simulink model "EHB_speedgoat_R2020a_V1"  (R2020a)
settings: Solver=FixedStepDiscrete  StartTime=0.0  StopTime=inf  FixedStep=0.001  RelTol=1e-3  EnableMultiTasking=on
model workspace (MAT data in the model file):
  A : Simulink.Signal (value not decoded)
  B : Simulink.Signal (value not decoded)
  C : Simulink.Signal (value not decoded)
  D : Simulink.Signal (value not decoded)
  E : Simulink.Signal (value not decoded)
  calin = [-9.96 -7.98 -5.98 -3.99 -1.994 0 1.995 3.992 5.99 7.98 9.97]
  calout = [-10 -8 -6 -4 -2 0 2 4 6 8 10]
symbols that are objects in the model workspace (value not decoded): C, D
undefined symbols (not defined in the file): Com1, none, ts_IO612
libraries: simulink x1436, xpcethercatlib x1223, yisutbxlib_utilities x256, xpcutilitieslib x156, hdlsllib x145, canmsglib x46, speedgoatlib_IO602_4 x11, speedgoatlib_IO611 x7, slrttcplib x4, CanManageLib x3, slrtlib x3, xpcseriallib x2
(part 5 of 30)

== system EHB_speedgoat_R2020a_V1/TIF_04/CB2020_3/Sw6 ==
  In2 : Inport
  In3 : Inport  Port=2
  Vol : Inport  Port=3
  Add : Sum
  Add1 : Sum
  Constant : Constant  Value=0.02
  Constant1 : Constant  Value=0.01
  Switch : Switch  Criteria=u2 > Threshold  Threshold=2.2
  Out1 : Outport
  wires:
  Constant/1 -> Add/2
  Add/1 -> Switch/3
  Add1/1 -> Switch/1
  Switch/1 -> Out1/1
  In3/1 -> Add/1
  In2/1 -> Switch/2
  Constant1/1 -> Add1/1
  Vol/1 -> Add1/2

== system EHB_speedgoat_R2020a_V1/TIF_04/CB2020_3/Sw7 ==
  In2 : Inport
  In3 : Inport  Port=2
  Vol : Inport  Port=3
  Add : Sum
  Add1 : Sum
  Constant : Constant  Value=0.02
  Constant1 : Constant  Value=0.01
  Switch : Switch  Criteria=u2 > Threshold  Threshold=2.2
  Out1 : Outport
  wires:
  In2/1 -> Switch/2
  In3/1 -> Add/1
  Switch/1 -> Out1/1
  Add1/1 -> Switch/1
  Add/1 -> Switch/3
  Constant/1 -> Add/2
  Constant1/1 -> Add1/1
  Vol/1 -> Add1/2

== system EHB_speedgoat_R2020a_V1/TIF_04/CB2020_3/Sw8 ==
  Vol : Inport
  In2 : Inport  Port=2
  In3 : Inport  Port=3
  Add : Sum
  Add1 : Sum
  Constant : Constant  Value=0.02
  Constant1 : Constant  Value=0.01
  Switch : Switch  Criteria=u2 > Threshold  Threshold=2.2
  Out1 : Outport
  wires:
  Constant/1 -> Add/2
  Add/1 -> Switch/3
  Switch/1 -> Out1/1
  In3/1 -> Add/1
  In2/1 -> Switch/2
  Constant1/1 -> Add1/1
  Vol/1 -> Add1/2
  Add1/1 -> Switch/1

== system EHB_speedgoat_R2020a_V1/TIF_04/CB2020_3/Sw9 ==
  In2 : Inport
  In3 : Inport  Port=2
  Vol : Inport  Port=3
  Add : Sum
  Add1 : Sum
  Constant : Constant  Value=0.02
  Constant1 : Constant  Value=0.01
  Switch : Switch  Criteria=u2 > Threshold  Threshold=2.2
  Out1 : Outport
  wires:
  In2/1 -> Switch/2
  In3/1 -> Add/1
  Switch/1 -> Out1/1
  Add1/1 -> Switch/1
  Add/1 -> Switch/3
  Constant/1 -> Add/2
  Constant1/1 -> Add1/1
  Vol/1 -> Add1/2

== system EHB_speedgoat_R2020a_V1/TIF_04/CB2020_3/mean1 ==
  In1 : Inport
  Add : Sum
  Add1 : Sum  Inputs=++++++++++++++++++++
  Add2 : Sum  Inputs=++++++++++++++++++++
  Delay{,1..39} (40 alike) : Delay  DelayLength=1
  Gain : Gain  Gain=1/40
  Vol : Outport
  wires:
  Add/1 -> Gain/1
  Gain/1 -> Vol/1
  Delay36/1 -> Delay37/1, Add2/7
  Delay37/1 -> Delay38/1, Add2/8
  Delay34/1 -> Delay35/1, Add2/5
  Delay33/1 -> Delay34/1, Add2/4
  Delay20/1 -> Delay21/1, Add2/1
  Delay32/1 -> Delay33/1, Add2/3
  Add2/1 -> Add/2
  Delay35/1 -> Delay36/1, Add2/6
  Delay21/1 -> Delay32/1, Add2/2
  Delay38/1 -> Delay39/1, Add2/9
  Delay39/1 -> Delay22/1, Add2/10
  Delay31/1 -> Add2/20
  Delay19/1 -> Add1/20, Delay20/1
  Delay30/1 -> Delay31/1, Add2/19
  Delay23/1 -> Delay24/1, Add2/12
  Delay27/1 -> Delay28/1, Add2/16
  Delay24/1 -> Delay25/1, Add2/13
  Delay22/1 -> Delay23/1, Add2/11
  Delay25/1 -> Delay26/1, Add2/14
  Delay26/1 -> Delay27/1, Add2/15
  Delay29/1 -> Delay30/1, Add2/18
  Delay28/1 -> Delay29/1, Add2/17
  Delay16/1 -> Add1/17, Delay17/1
  Delay17/1 -> Add1/18, Delay18/1
  Delay14/1 -> Add1/15, Delay15/1
  Delay13/1 -> Add1/14, Delay14/1
  Delay10/1 -> Add1/11, Delay11/1
  Delay12/1 -> Add1/13, Delay13/1
  Delay15/1 -> Add1/16, Delay16/1
  Delay11/1 -> Add1/12, Delay12/1
  Delay18/1 -> Add1/19, Delay19/1
  In1/1 -> Delay/1
  Delay9/1 -> Add1/10, Delay10/1
  Delay8/1 -> Add1/9, Delay9/1
  Delay1/1 -> Add1/2, Delay2/1
  Delay5/1 -> Add1/6, Delay6/1
  Add1/1 -> Add/1
  Delay2/1 -> Add1/3, Delay3/1
  Delay/1 -> Add1/1, Delay1/1
  Delay3/1 -> Add1/4, Delay4/1
  Delay4/1 -> Add1/5, Delay5/1
  Delay7/1 -> Add1/8, Delay8/1
  Delay6/1 -> Add1/7, Delay7/1

== system EHB_speedgoat_R2020a_V1/TIF_04/CB2020_3/mean10 ==
  In1 : Inport
  Add : Sum
  Add1 : Sum  Inputs=++++++++++++++++++++
  Add2 : Sum  Inputs=++++++++++++++++++++
  Delay{,1..39} (40 alike) : Delay  DelayLength=1
  Gain : Gain  Gain=1/40
  Vol : Outport
  wires:
  Delay6/1 -> Delay7/1, Add1/7
  Delay7/1 -> Delay8/1, Add1/8
  Delay4/1 -> Delay5/1, Add1/5
  Delay3/1 -> Delay4/1, Add1/4
  Delay/1 -> Delay1/1, Add1/1
  Delay2/1 -> Delay3/1, Add1/3
  Add1/1 -> Add/1
  Delay5/1 -> Delay6/1, Add1/6
  Delay1/1 -> Delay2/1, Add1/2
  Delay8/1 -> Delay9/1, Add1/9
  Delay9/1 -> Delay10/1, Add1/10
  In1/1 -> Delay/1
  Delay18/1 -> Delay19/1, Add1/19
  Delay11/1 -> Delay12/1, Add1/12
  Delay15/1 -> Delay16/1, Add1/16
  Delay12/1 -> Delay13/1, Add1/13
  Delay10/1 -> Delay11/1, Add1/11
  Delay13/1 -> Delay14/1, Add1/14
  Delay14/1 -> Delay15/1, Add1/15
  Delay17/1 -> Delay18/1, Add1/18
  Delay16/1 -> Delay17/1, Add1/17
  Delay28/1 -> Add2/17, Delay29/1
  Delay29/1 -> Add2/18, Delay30/1
  Delay26/1 -> Add2/15, Delay27/1
  Delay25/1 -> Add2/14, Delay26/1
  Delay22/1 -> Add2/11, Delay23/1
  Delay24/1 -> Add2/13, Delay25/1
  Delay27/1 -> Add2/16, Delay28/1
  Delay23/1 -> Add2/12, Delay24/1
  Delay30/1 -> Add2/19, Delay31/1
  Delay19/1 -> Delay20/1, Add1/20
  Delay31/1 -> Add2/20
  Delay39/1 -> Add2/10, Delay22/1
  Delay38/1 -> Add2/9, Delay39/1
  Delay21/1 -> Add2/2, Delay32/1
  Delay35/1 -> Add2/6, Delay36/1
  Add2/1 -> Add/2
  Delay32/1 -> Add2/3, Delay33/1
  Delay20/1 -> Add2/1, Delay21/1
  Delay33/1 -> Add2/4, Delay34/1
  Delay34/1 -> Add2/5, Delay35/1
  Delay37/1 -> Add2/8, Delay38/1
  Delay36/1 -> Add2/7, Delay37/1
  Gain/1 -> Vol/1
  Add/1 -> Gain/1

== system EHB_speedgoat_R2020a_V1/TIF_04/CB2020_3/mean11 ==
  In1 : Inport
  Add : Sum
  Add1 : Sum  Inputs=++++++++++++++++++++
  Add2 : Sum  Inputs=++++++++++++++++++++
  Delay{,1..39} (40 alike) : Delay  DelayLength=1
  Gain : Gain  Gain=1/40
  Vol : Outport
  wires:
  Add/1 -> Gain/1
  Gain/1 -> Vol/1
  Delay36/1 -> Delay37/1, Add2/7
  Delay37/1 -> Delay38/1, Add2/8
  Delay34/1 -> Delay35/1, Add2/5
  Delay33/1 -> Delay34/1, Add2/4
  Delay20/1 -> Delay21/1, Add2/1
  Delay32/1 -> Delay33/1, Add2/3
  Add2/1 -> Add/2
  Delay35/1 -> Delay36/1, Add2/6
  Delay21/1 -> Delay32/1, Add2/2
  Delay38/1 -> Delay39/1, Add2/9
  Delay39/1 -> Delay22/1, Add2/10
  Delay31/1 -> Add2/20
  Delay19/1 -> Add1/20, Delay20/1
  Delay30/1 -> Delay31/1, Add2/19
  Delay23/1 -> Delay24/1, Add2/12
  Delay27/1 -> Delay28/1, Add2/16
  Delay24/1 -> Delay25/1, Add2/13
  Delay22/1 -> Delay23/1, Add2/11
  Delay25/1 -> Delay26/1, Add2/14
  Delay26/1 -> Delay27/1, Add2/15
  Delay29/1 -> Delay30/1, Add2/18
  Delay28/1 -> Delay29/1, Add2/17
  Delay16/1 -> Add1/17, Delay17/1
  Delay17/1 -> Add1/18, Delay18/1
  Delay14/1 -> Add1/15, Delay15/1
  Delay13/1 -> Add1/14, Delay14/1
  Delay10/1 -> Add1/11, Delay11/1
  Delay12/1 -> Add1/13, Delay13/1
  Delay15/1 -> Add1/16, Delay16/1
  Delay11/1 -> Add1/12, Delay12/1
  Delay18/1 -> Add1/19, Delay19/1
  In1/1 -> Delay/1
  Delay9/1 -> Add1/10, Delay10/1
  Delay8/1 -> Add1/9, Delay9/1
  Delay1/1 -> Add1/2, Delay2/1
  Delay5/1 -> Add1/6, Delay6/1
  Add1/1 -> Add/1
  Delay2/1 -> Add1/3, Delay3/1
  Delay/1 -> Add1/1, Delay1/1
  Delay3/1 -> Add1/4, Delay4/1
  Delay4/1 -> Add1/5, Delay5/1
  Delay7/1 -> Add1/8, Delay8/1
  Delay6/1 -> Add1/7, Delay7/1

== system EHB_speedgoat_R2020a_V1/TIF_04/CB2020_3/mean12 ==
  In1 : Inport
  Add : Sum
  Add1 : Sum  Inputs=++++++++++++++++++++
  Add2 : Sum  Inputs=++++++++++++++++++++
  Delay{,1..39} (40 alike) : Delay  DelayLength=1
  Gain : Gain  Gain=1/40
  Vol : Outport
  wires:
  Delay6/1 -> Delay7/1, Add1/7
  Delay7/1 -> Delay8/1, Add1/8
  Delay4/1 -> Delay5/1, Add1/5
  Delay3/1 -> Delay4/1, Add1/4
  Delay/1 -> Delay1/1, Add1/1
  Delay2/1 -> Delay3/1, Add1/3
  Add1/1 -> Add/1
  Delay5/1 -> Delay6/1, Add1/6
  Delay1/1 -> Delay2/1, Add1/2
  Delay8/1 -> Delay9/1, Add1/9
  Delay9/1 -> Delay10/1, Add1/10
  In1/1 -> Delay/1
  Delay18/1 -> Delay19/1, Add1/19
  Delay11/1 -> Delay12/1, Add1/12
  Delay15/1 -> Delay16/1, Add1/16
  Delay12/1 -> Delay13/1, Add1/13
  Delay10/1 -> Delay11/1, Add1/11
  Delay13/1 -> Delay14/1, Add1/14
  Delay14/1 -> Delay15/1, Add1/15
  Delay17/1 -> Delay18/1, Add1/18
  Delay16/1 -> Delay17/1, Add1/17
  Delay28/1 -> Add2/17, Delay29/1
  Delay29/1 -> Add2/18, Delay30/1
  Delay26/1 -> Add2/15, Delay27/1
  Delay25/1 -> Add2/14, Delay26/1
  Delay22/1 -> Add2/11, Delay23/1
  Delay24/1 -> Add2/13, Delay25/1
  Delay27/1 -> Add2/16, Delay28/1
  Delay23/1 -> Add2/12, Delay24/1
  Delay30/1 -> Add2/19, Delay31/1
  Delay19/1 -> Delay20/1, Add1/20
  Delay31/1 -> Add2/20
  Delay39/1 -> Add2/10, Delay22/1
  Delay38/1 -> Add2/9, Delay39/1
  Delay21/1 -> Add2/2, Delay32/1
  Delay35/1 -> Add2/6, Delay36/1
  Add2/1 -> Add/2
  Delay32/1 -> Add2/3, Delay33/1
  Delay20/1 -> Add2/1, Delay21/1
  Delay33/1 -> Add2/4, Delay34/1
  Delay34/1 -> Add2/5, Delay35/1
  Delay37/1 -> Add2/8, Delay38/1
  Delay36/1 -> Add2/7, Delay37/1
  Gain/1 -> Vol/1
  Add/1 -> Gain/1

== system EHB_speedgoat_R2020a_V1/TIF_04/CB2020_3/mean13 ==
  In1 : Inport
  Add : Sum  Inputs=++++
  Add{1..4} (4 alike) : Sum  Inputs=++++++++++++++++++++
  Delay{,1..79} (80 alike) : Delay  DelayLength=1
  Gain : Gain  Gain=1/80
  Vol : Outport
  wires:
  Add/1 -> Gain/1
  Gain/1 -> Vol/1
  Delay36/1 -> Delay37/1, Add2/7
  Delay37/1 -> Delay38/1, Add2/8
  Delay34/1 -> Delay35/1, Add2/5
  Delay33/1 -> Delay34/1, Add2/4
  Delay20/1 -> Delay21/1, Add2/1
  Delay32/1 -> Delay33/1, Add2/3
  Add2/1 -> Add/2
  Delay35/1 -> Delay36/1, Add2/6
  Delay21/1 -> Delay32/1, Add2/2
  Delay38/1 -> Delay39/1, Add2/9
  Delay39/1 -> Delay22/1, Add2/10
  Delay19/1 -> Add1/20, Delay20/1
  Delay30/1 -> Delay31/1, Add2/19
  Delay23/1 -> Delay24/1, Add2/12
  Delay27/1 -> Delay28/1, Add2/16
  Delay24/1 -> Delay25/1, Add2/13
  Delay22/1 -> Delay23/1, Add2/11
  Delay25/1 -> Delay26/1, Add2/14
  Delay26/1 -> Delay27/1, Add2/15
  Delay29/1 -> Delay30/1, Add2/18
  Delay28/1 -> Delay29/1, Add2/17
  Delay16/1 -> Add1/17, Delay17/1
  Delay17/1 -> Add1/18, Delay18/1
  Delay14/1 -> Add1/15, Delay15/1
  Delay13/1 -> Add1/14, Delay14/1
  Delay10/1 -> Add1/11, Delay11/1
  Delay12/1 -> Add1/13, Delay13/1
  Delay15/1 -> Add1/16, Delay16/1
  Delay11/1 -> Add1/12, Delay12/1
  Delay18/1 -> Add1/19, Delay19/1
  In1/1 -> Delay/1
  Delay9/1 -> Add1/10, Delay10/1
  Delay8/1 -> Add1/9, Delay9/1
  Delay1/1 -> Add1/2, Delay2/1
  Delay5/1 -> Add1/6, Delay6/1
  Add1/1 -> Add/1
  Delay2/1 -> Add1/3, Delay3/1
  Delay/1 -> Add1/1, Delay1/1
  Delay3/1 -> Add1/4, Delay4/1
  Delay4/1 -> Add1/5, Delay5/1
  Delay7/1 -> Add1/8, Delay8/1
  Delay6/1 -> Add1/7, Delay7/1
  Delay48/1 -> Add3/17, Delay49/1
  Delay49/1 -> Add3/18, Delay50/1
  Delay46/1 -> Add3/15, Delay47/1
  Delay45/1 -> Add3/14, Delay46/1
  Delay42/1 -> Add3/11, Delay43/1
  Delay44/1 -> Add3/13, Delay45/1
  Delay47/1 -> Add3/16, Delay48/1
  Delay43/1 -> Add3/12, Delay44/1
  Delay50/1 -> Add3/19, Delay51/1
  Delay31/1 -> Delay40/1, Add2/20
  Delay59/1 -> Add3/10, Delay42/1
  Delay58/1 -> Add3/9, Delay59/1
  Delay41/1 -> Add3/2, Delay52/1
  Delay55/1 -> Add3/6, Delay56/1
  Add3/1 -> Add/3
  Delay52/1 -> Add3/3, Delay53/1
  Delay40/1 -> Add3/1, Delay41/1
  Delay53/1 -> Add3/4, Delay54/1
  Delay54/1 -> Add3/5, Delay55/1
  Delay57/1 -> Add3/8, Delay58/1
  Delay56/1 -> Add3/7, Delay57/1
  Delay76/1 -> Delay77/1, Add4/7
  Delay77/1 -> Delay78/1, Add4/8
  Delay74/1 -> Delay75/1, Add4/5
  Delay73/1 -> Delay74/1, Add4/4
  Delay60/1 -> Delay61/1, Add4/1
  Delay72/1 -> Delay73/1, Add4/3
  Add4/1 -> Add/4
  Delay75/1 -> Delay76/1, Add4/6
  Delay61/1 -> Delay72/1, Add4/2
  Delay78/1 -> Delay79/1, Add4/9
  Delay79/1 -> Delay62/1, Add4/10
  Delay71/1 -> Add4/20
  Delay51/1 -> Delay60/1, Add3/20
  Delay70/1 -> Delay71/1, Add4/19
  Delay63/1 -> Delay64/1, Add4/12
  Delay67/1 -> Delay68/1, Add4/16
  Delay64/1 -> Delay65/1, Add4/13
  Delay62/1 -> Delay63/1, Add4/11
  Delay65/1 -> Delay66/1, Add4/14
  Delay66/1 -> Delay67/1, Add4/15
  Delay69/1 -> Delay70/1, Add4/18
  Delay68/1 -> Delay69/1, Add4/17

== system EHB_speedgoat_R2020a_V1/TIF_04/CB2020_3/mean14 ==
  In1 : Inport
  Add : Sum  Inputs=++++
  Add{1..4} (4 alike) : Sum  Inputs=++++++++++++++++++++
  Delay{,1..79} (80 alike) : Delay  DelayLength=1
  Gain : Gain  Gain=1/80
  Vol : Outport
  wires:
  Delay68/1 -> Add4/17, Delay69/1
  Delay69/1 -> Add4/18, Delay70/1
  Delay66/1 -> Add4/15, Delay67/1
  Delay65/1 -> Add4/14, Delay66/1
  Delay62/1 -> Add4/11, Delay63/1
  Delay64/1 -> Add4/13, Delay65/1
  Delay67/1 -> Add4/16, Delay68/1
  Delay63/1 -> Add4/12, Delay64/1
  Delay70/1 -> Add4/19, Delay71/1
  Delay51/1 -> Add3/20, Delay60/1
  Delay71/1 -> Add4/20
  Delay79/1 -> Add4/10, Delay62/1
  Delay78/1 -> Add4/9, Delay79/1
  Delay61/1 -> Add4/2, Delay72/1
  Delay75/1 -> Add4/6, Delay76/1
  Add4/1 -> Add/4
  Delay72/1 -> Add4/3, Delay73/1
  Delay60/1 -> Add4/1, Delay61/1
  Delay73/1 -> Add4/4, Delay74/1
  Delay74/1 -> Add4/5, Delay75/1
  Delay77/1 -> Add4/8, Delay78/1
  Delay76/1 -> Add4/7, Delay77/1
  Delay56/1 -> Delay57/1, Add3/7
  Delay57/1 -> Delay58/1, Add3/8
  Delay54/1 -> Delay55/1, Add3/5
  Delay53/1 -> Delay54/1, Add3/4
  Delay40/1 -> Delay41/1, Add3/1
  Delay52/1 -> Delay53/1, Add3/3
  Add3/1 -> Add/3
  Delay55/1 -> Delay56/1, Add3/6
  Delay41/1 -> Delay52/1, Add3/2
  Delay58/1 -> Delay59/1, Add3/9
  Delay59/1 -> Delay42/1, Add3/10
  Delay31/1 -> Add2/20, Delay40/1
  Delay50/1 -> Delay51/1, Add3/19
  Delay43/1 -> Delay44/1, Add3/12
  Delay47/1 -> Delay48/1, Add3/16
  Delay44/1 -> Delay45/1, Add3/13
  Delay42/1 -> Delay43/1, Add3/11
  Delay45/1 -> Delay46/1, Add3/14
  Delay46/1 -> Delay47/1, Add3/15
  Delay49/1 -> Delay50/1, Add3/18
  Delay48/1 -> Delay49/1, Add3/17
  Delay6/1 -> Delay7/1, Add1/7
  Delay7/1 -> Delay8/1, Add1/8
  Delay4/1 -> Delay5/1, Add1/5
  Delay3/1 -> Delay4/1, Add1/4
  Delay/1 -> Delay1/1, Add1/1
  Delay2/1 -> Delay3/1, Add1/3
  Add1/1 -> Add/1
  Delay5/1 -> Delay6/1, Add1/6
  Delay1/1 -> Delay2/1, Add1/2
  Delay8/1 -> Delay9/1, Add1/9
  Delay9/1 -> Delay10/1, Add1/10
  In1/1 -> Delay/1
  Delay18/1 -> Delay19/1, Add1/19
  Delay11/1 -> Delay12/1, Add1/12
  Delay15/1 -> Delay16/1, Add1/16
  Delay12/1 -> Delay13/1, Add1/13
  Delay10/1 -> Delay11/1, Add1/11
  Delay13/1 -> Delay14/1, Add1/14
  Delay14/1 -> Delay15/1, Add1/15
  Delay17/1 -> Delay18/1, Add1/18
  Delay16/1 -> Delay17/1, Add1/17
  Delay28/1 -> Add2/17, Delay29/1
  Delay29/1 -> Add2/18, Delay30/1
  Delay26/1 -> Add2/15, Delay27/1
  Delay25/1 -> Add2/14, Delay26/1
  Delay22/1 -> Add2/11, Delay23/1
  Delay24/1 -> Add2/13, Delay25/1
  Delay27/1 -> Add2/16, Delay28/1
  Delay23/1 -> Add2/12, Delay24/1
  Delay30/1 -> Add2/19, Delay31/1
  Delay19/1 -> Delay20/1, Add1/20
  Delay39/1 -> Add2/10, Delay22/1
  Delay38/1 -> Add2/9, Delay39/1
  Delay21/1 -> Add2/2, Delay32/1
  Delay35/1 -> Add2/6, Delay36/1
  Add2/1 -> Add/2
  Delay32/1 -> Add2/3, Delay33/1
  Delay20/1 -> Add2/1, Delay21/1
  Delay33/1 -> Add2/4, Delay34/1
  Delay34/1 -> Add2/5, Delay35/1
  Delay37/1 -> Add2/8, Delay38/1
  Delay36/1 -> Add2/7, Delay37/1
  Gain/1 -> Vol/1
  Add/1 -> Gain/1

== system EHB_speedgoat_R2020a_V1/TIF_04/CB2020_3/mean15 ==
  In1 : Inport
  Add : Sum  Inputs=++++
  Add{1..4} (4 alike) : Sum  Inputs=++++++++++++++++++++
  Delay{,1..79} (80 alike) : Delay  DelayLength=1
  Gain : Gain  Gain=1/80
  Vol : Outport
  wires:
  Add/1 -> Gain/1
  Gain/1 -> Vol/1
  Delay36/1 -> Delay37/1, Add2/7
  Delay37/1 -> Delay38/1, Add2/8
  Delay34/1 -> Delay35/1, Add2/5
  Delay33/1 -> Delay34/1, Add2/4
  Delay20/1 -> Delay21/1, Add2/1
  Delay32/1 -> Delay33/1, Add2/3
  Add2/1 -> Add/2
  Delay35/1 -> Delay36/1, Add2/6
  Delay21/1 -> Delay32/1, Add2/2
  Delay38/1 -> Delay39/1, Add2/9
  Delay39/1 -> Delay22/1, Add2/10
  Delay19/1 -> Add1/20, Delay20/1
  Delay30/1 -> Delay31/1, Add2/19
  Delay23/1 -> Delay24/1, Add2/12
  Delay27/1 -> Delay28/1, Add2/16
  Delay24/1 -> Delay25/1, Add2/13
  Delay22/1 -> Delay23/1, Add2/11
  Delay25/1 -> Delay26/1, Add2/14
  Delay26/1 -> Delay27/1, Add2/15
  Delay29/1 -> Delay30/1, Add2/18
  Delay28/1 -> Delay29/1, Add2/17
  Delay16/1 -> Add1/17, Delay17/1
  Delay17/1 -> Add1/18, Delay18/1
  Delay14/1 -> Add1/15, Delay15/1
  Delay13/1 -> Add1/14, Delay14/1
  Delay10/1 -> Add1/11, Delay11/1
  Delay12/1 -> Add1/13, Delay13/1
  Delay15/1 -> Add1/16, Delay16/1
  Delay11/1 -> Add1/12, Delay12/1
  Delay18/1 -> Add1/19, Delay19/1
  In1/1 -> Delay/1
  Delay9/1 -> Add1/10, Delay10/1
  Delay8/1 -> Add1/9, Delay9/1
  Delay1/1 -> Add1/2, Delay2/1
  Delay5/1 -> Add1/6, Delay6/1
  Add1/1 -> Add/1
  Delay2/1 -> Add1/3, Delay3/1
  Delay/1 -> Add1/1, Delay1/1
  Delay3/1 -> Add1/4, Delay4/1
  Delay4/1 -> Add1/5, Delay5/1
  Delay7/1 -> Add1/8, Delay8/1
  Delay6/1 -> Add1/7, Delay7/1
  Delay48/1 -> Add3/17, Delay49/1
  Delay49/1 -> Add3/18, Delay50/1
  Delay46/1 -> Add3/15, Delay47/1
  Delay45/1 -> Add3/14, Delay46/1
  Delay42/1 -> Add3/11, Delay43/1
  Delay44/1 -> Add3/13, Delay45/1
  Delay47/1 -> Add3/16, Delay48/1
  Delay43/1 -> Add3/12, Delay44/1
  Delay50/1 -> Add3/19, Delay51/1
  Delay31/1 -> Delay40/1, Add2/20
  Delay59/1 -> Add3/10, Delay42/1
  Delay58/1 -> Add3/9, Delay59/1
  Delay41/1 -> Add3/2, Delay52/1
  Delay55/1 -> Add3/6, Delay56/1
  Add3/1 -> Add/3
  Delay52/1 -> Add3/3, Delay53/1
  Delay40/1 -> Add3/1, Delay41/1
  Delay53/1 -> Add3/4, Delay54/1
  Delay54/1 -> Add3/5, Delay55/1
  Delay57/1 -> Add3/8, Delay58/1
  Delay56/1 -> Add3/7, Delay57/1
  Delay76/1 -> Delay77/1, Add4/7
  Delay77/1 -> Delay78/1, Add4/8
  Delay74/1 -> Delay75/1, Add4/5
  Delay73/1 -> Delay74/1, Add4/4
  Delay60/1 -> Delay61/1, Add4/1
  Delay72/1 -> Delay73/1, Add4/3
  Add4/1 -> Add/4
  Delay75/1 -> Delay76/1, Add4/6
  Delay61/1 -> Delay72/1, Add4/2
  Delay78/1 -> Delay79/1, Add4/9
  Delay79/1 -> Delay62/1, Add4/10
  Delay71/1 -> Add4/20
  Delay51/1 -> Delay60/1, Add3/20
  Delay70/1 -> Delay71/1, Add4/19
  Delay63/1 -> Delay64/1, Add4/12
  Delay67/1 -> Delay68/1, Add4/16
  Delay64/1 -> Delay65/1, Add4/13
  Delay62/1 -> Delay63/1, Add4/11
  Delay65/1 -> Delay66/1, Add4/14
  Delay66/1 -> Delay67/1, Add4/15
  Delay69/1 -> Delay70/1, Add4/18
  Delay68/1 -> Delay69/1, Add4/17

== system EHB_speedgoat_R2020a_V1/TIF_04/CB2020_3/mean16 ==
  In1 : Inport
  Add : Sum  Inputs=++++
  Add{1..4} (4 alike) : Sum  Inputs=++++++++++++++++++++
  Delay{,1..79} (80 alike) : Delay  DelayLength=1
  Gain : Gain  Gain=1/80
  Vol : Outport
  wires:
  Delay68/1 -> Add4/17, Delay69/1
  Delay69/1 -> Add4/18, Delay70/1
  Delay66/1 -> Add4/15, Delay67/1
  Delay65/1 -> Add4/14, Delay66/1
  Delay62/1 -> Add4/11, Delay63/1
  Delay64/1 -> Add4/13, Delay65/1
  Delay67/1 -> Add4/16, Delay68/1
  Delay63/1 -> Add4/12, Delay64/1
  Delay70/1 -> Add4/19, Delay71/1
  Delay51/1 -> Add3/20, Delay60/1
  Delay71/1 -> Add4/20
  Delay79/1 -> Add4/10, Delay62/1
  Delay78/1 -> Add4/9, Delay79/1
  Delay61/1 -> Add4/2, Delay72/1
  Delay75/1 -> Add4/6, Delay76/1
  Add4/1 -> Add/4
  Delay72/1 -> Add4/3, Delay73/1
  Delay60/1 -> Add4/1, Delay61/1
  Delay73/1 -> Add4/4, Delay74/1
  Delay74/1 -> Add4/5, Delay75/1
  Delay77/1 -> Add4/8, Delay78/1
  Delay76/1 -> Add4/7, Delay77/1
  Delay56/1 -> Delay57/1, Add3/7
  Delay57/1 -> Delay58/1, Add3/8
  Delay54/1 -> Delay55/1, Add3/5
  Delay53/1 -> Delay54/1, Add3/4
  Delay40/1 -> Delay41/1, Add3/1
  Delay52/1 -> Delay53/1, Add3/3
  Add3/1 -> Add/3
  Delay55/1 -> Delay56/1, Add3/6
  Delay41/1 -> Delay52/1, Add3/2
  Delay58/1 -> Delay59/1, Add3/9
  Delay59/1 -> Delay42/1, Add3/10
  Delay31/1 -> Add2/20, Delay40/1
  Delay50/1 -> Delay51/1, Add3/19
  Delay43/1 -> Delay44/1, Add3/12
  Delay47/1 -> Delay48/1, Add3/16
  Delay44/1 -> Delay45/1, Add3/13
  Delay42/1 -> Delay43/1, Add3/11
  Delay45/1 -> Delay46/1, Add3/14
  Delay46/1 -> Delay47/1, Add3/15
  Delay49/1 -> Delay50/1, Add3/18
  Delay48/1 -> Delay49/1, Add3/17
  Delay6/1 -> Delay7/1, Add1/7
  Delay7/1 -> Delay8/1, Add1/8
  Delay4/1 -> Delay5/1, Add1/5
  Delay3/1 -> Delay4/1, Add1/4
  Delay/1 -> Delay1/1, Add1/1
  Delay2/1 -> Delay3/1, Add1/3
  Add1/1 -> Add/1
  Delay5/1 -> Delay6/1, Add1/6
  Delay1/1 -> Delay2/1, Add1/2
  Delay8/1 -> Delay9/1, Add1/9
  Delay9/1 -> Delay10/1, Add1/10
  In1/1 -> Delay/1
  Delay18/1 -> Delay19/1, Add1/19
  Delay11/1 -> Delay12/1, Add1/12
  Delay15/1 -> Delay16/1, Add1/16
  Delay12/1 -> Delay13/1, Add1/13
  Delay10/1 -> Delay11/1, Add1/11
  Delay13/1 -> Delay14/1, Add1/14
  Delay14/1 -> Delay15/1, Add1/15
  Delay17/1 -> Delay18/1, Add1/18
  Delay16/1 -> Delay17/1, Add1/17
  Delay28/1 -> Add2/17, Delay29/1
  Delay29/1 -> Add2/18, Delay30/1
  Delay26/1 -> Add2/15, Delay27/1
  Delay25/1 -> Add2/14, Delay26/1
  Delay22/1 -> Add2/11, Delay23/1
  Delay24/1 -> Add2/13, Delay25/1
  Delay27/1 -> Add2/16, Delay28/1
  Delay23/1 -> Add2/12, Delay24/1
  Delay30/1 -> Add2/19, Delay31/1
  Delay19/1 -> Delay20/1, Add1/20
  Delay39/1 -> Add2/10, Delay22/1
  Delay38/1 -> Add2/9, Delay39/1
  Delay21/1 -> Add2/2, Delay32/1
  Delay35/1 -> Add2/6, Delay36/1
  Add2/1 -> Add/2
  Delay32/1 -> Add2/3, Delay33/1
  Delay20/1 -> Add2/1, Delay21/1
  Delay33/1 -> Add2/4, Delay34/1
  Delay34/1 -> Add2/5, Delay35/1
  Delay37/1 -> Add2/8, Delay38/1
  Delay36/1 -> Add2/7, Delay37/1
  Gain/1 -> Vol/1
  Add/1 -> Gain/1

== system EHB_speedgoat_R2020a_V1/TIF_04/CB2020_3/mean2 ==
  In1 : Inport
  Add : Sum
  Add1 : Sum  Inputs=++++++++++++++++++++
  Add2 : Sum  Inputs=++++++++++++++++++++
  Delay{,1..39} (40 alike) : Delay  DelayLength=1
  Gain : Gain  Gain=1/40
  Vol : Outport
  wires:
  Delay6/1 -> Delay7/1, Add1/7
  Delay7/1 -> Delay8/1, Add1/8
  Delay4/1 -> Delay5/1, Add1/5
  Delay3/1 -> Delay4/1, Add1/4
  Delay/1 -> Delay1/1, Add1/1
  Delay2/1 -> Delay3/1, Add1/3
  Add1/1 -> Add/1
  Delay5/1 -> Delay6/1, Add1/6
  Delay1/1 -> Delay2/1, Add1/2
  Delay8/1 -> Delay9/1, Add1/9
  Delay9/1 -> Delay10/1, Add1/10
  In1/1 -> Delay/1
  Delay18/1 -> Delay19/1, Add1/19
  Delay11/1 -> Delay12/1, Add1/12
  Delay15/1 -> Delay16/1, Add1/16
  Delay12/1 -> Delay13/1, Add1/13
  Delay10/1 -> Delay11/1, Add1/11
  Delay13/1 -> Delay14/1, Add1/14
  Delay14/1 -> Delay15/1, Add1/15
  Delay17/1 -> Delay18/1, Add1/18
  Delay16/1 -> Delay17/1, Add1/17
  Delay28/1 -> Add2/17, Delay29/1
  Delay29/1 -> Add2/18, Delay30/1
  Delay26/1 -> Add2/15, Delay27/1
  Delay25/1 -> Add2/14, Delay26/1
  Delay22/1 -> Add2/11, Delay23/1
  Delay24/1 -> Add2/13, Delay25/1
  Delay27/1 -> Add2/16, Delay28/1
  Delay23/1 -> Add2/12, Delay24/1
  Delay30/1 -> Add2/19, Delay31/1
  Delay19/1 -> Delay20/1, Add1/20
  Delay31/1 -> Add2/20
  Delay39/1 -> Add2/10, Delay22/1
  Delay38/1 -> Add2/9, Delay39/1
  Delay21/1 -> Add2/2, Delay32/1
  Delay35/1 -> Add2/6, Delay36/1
  Add2/1 -> Add/2
  Delay32/1 -> Add2/3, Delay33/1
  Delay20/1 -> Add2/1, Delay21/1
  Delay33/1 -> Add2/4, Delay34/1
  Delay34/1 -> Add2/5, Delay35/1
  Delay37/1 -> Add2/8, Delay38/1
  Delay36/1 -> Add2/7, Delay37/1
  Gain/1 -> Vol/1
  Add/1 -> Gain/1

== system EHB_speedgoat_R2020a_V1/TIF_04/CB2020_3/mean3 ==
  In1 : Inport
  Add : Sum
  Add1 : Sum  Inputs=++++++++++++++++++++
  Add2 : Sum  Inputs=++++++++++++++++++++
  Delay{,1..39} (40 alike) : Delay  DelayLength=1
  Gain : Gain  Gain=1/40
  Vol : Outport
  wires:
  Add/1 -> Gain/1
  Gain/1 -> Vol/1
  Delay36/1 -> Delay37/1, Add2/7
  Delay37/1 -> Delay38/1, Add2/8
  Delay34/1 -> Delay35/1, Add2/5
  Delay33/1 -> Delay34/1, Add2/4
  Delay20/1 -> Delay21/1, Add2/1
  Delay32/1 -> Delay33/1, Add2/3
  Add2/1 -> Add/2
  Delay35/1 -> Delay36/1, Add2/6
  Delay21/1 -> Delay32/1, Add2/2
  Delay38/1 -> Delay39/1, Add2/9
  Delay39/1 -> Delay22/1, Add2/10
  Delay31/1 -> Add2/20
  Delay19/1 -> Add1/20, Delay20/1
  Delay30/1 -> Delay31/1, Add2/19
  Delay23/1 -> Delay24/1, Add2/12
  Delay27/1 -> Delay28/1, Add2/16
  Delay24/1 -> Delay25/1, Add2/13
  Delay22/1 -> Delay23/1, Add2/11
  Delay25/1 -> Delay26/1, Add2/14
  Delay26/1 -> Delay27/1, Add2/15
  Delay29/1 -> Delay30/1, Add2/18
  Delay28/1 -> Delay29/1, Add2/17
  Delay16/1 -> Add1/17, Delay17/1
  Delay17/1 -> Add1/18, Delay18/1
  Delay14/1 -> Add1/15, Delay15/1
  Delay13/1 -> Add1/14, Delay14/1
  Delay10/1 -> Add1/11, Delay11/1
  Delay12/1 -> Add1/13, Delay13/1
  Delay15/1 -> Add1/16, Delay16/1
  Delay11/1 -> Add1/12, Delay12/1
  Delay18/1 -> Add1/19, Delay19/1
  In1/1 -> Delay/1
  Delay9/1 -> Add1/10, Delay10/1
  Delay8/1 -> Add1/9, Delay9/1
  Delay1/1 -> Add1/2, Delay2/1
  Delay5/1 -> Add1/6, Delay6/1
  Add1/1 -> Add/1
  Delay2/1 -> Add1/3, Delay3/1
  Delay/1 -> Add1/1, Delay1/1
  Delay3/1 -> Add1/4, Delay4/1
  Delay4/1 -> Add1/5, Delay5/1
  Delay7/1 -> Add1/8, Delay8/1
  Delay6/1 -> Add1/7, Delay7/1

== system EHB_speedgoat_R2020a_V1/TIF_04/CB2020_3/mean4 ==
  In1 : Inport
  Add : Sum
  Add1 : Sum  Inputs=++++++++++++++++++++
  Add2 : Sum  Inputs=++++++++++++++++++++
  Delay{,1..39} (40 alike) : Delay  DelayLength=1
  Gain : Gain  Gain=1/40
  Vol : Outport
  wires:
  Delay6/1 -> Delay7/1, Add1/7
  Delay7/1 -> Delay8/1, Add1/8
  Delay4/1 -> Delay5/1, Add1/5
  Delay3/1 -> Delay4/1, Add1/4
  Delay/1 -> Delay1/1, Add1/1
  Delay2/1 -> Delay3/1, Add1/3
  Add1/1 -> Add/1
  Delay5/1 -> Delay6/1, Add1/6
  Delay1/1 -> Delay2/1, Add1/2
  Delay8/1 -> Delay9/1, Add1/9
  Delay9/1 -> Delay10/1, Add1/10
  In1/1 -> Delay/1
  Delay18/1 -> Delay19/1, Add1/19
  Delay11/1 -> Delay12/1, Add1/12
  Delay15/1 -> Delay16/1, Add1/16
  Delay12/1 -> Delay13/1, Add1/13
  Delay10/1 -> Delay11/1, Add1/11
  Delay13/1 -> Delay14/1, Add1/14
  Delay14/1 -> Delay15/1, Add1/15
  Delay17/1 -> Delay18/1, Add1/18
  Delay16/1 -> Delay17/1, Add1/17
  Delay28/1 -> Add2/17, Delay29/1
  Delay29/1 -> Add2/18, Delay30/1
  Delay26/1 -> Add2/15, Delay27/1
  Delay25/1 -> Add2/14, Delay26/1
  Delay22/1 -> Add2/11, Delay23/1
  Delay24/1 -> Add2/13, Delay25/1
  Delay27/1 -> Add2/16, Delay28/1
  Delay23/1 -> Add2/12, Delay24/1
  Delay30/1 -> Add2/19, Delay31/1
  Delay19/1 -> Delay20/1, Add1/20
  Delay31/1 -> Add2/20
  Delay39/1 -> Add2/10, Delay22/1
  Delay38/1 -> Add2/9, Delay39/1
  Delay21/1 -> Add2/2, Delay32/1
  Delay35/1 -> Add2/6, Delay36/1
  Add2/1 -> Add/2
  Delay32/1 -> Add2/3, Delay33/1
  Delay20/1 -> Add2/1, Delay21/1
  Delay33/1 -> Add2/4, Delay34/1
  Delay34/1 -> Add2/5, Delay35/1
  Delay37/1 -> Add2/8, Delay38/1
  Delay36/1 -> Add2/7, Delay37/1
  Gain/1 -> Vol/1
  Add/1 -> Gain/1

== system EHB_speedgoat_R2020a_V1/TIF_04/CB2020_3/mean5 ==
  In1 : Inport
  Add : Sum
  Add1 : Sum  Inputs=++++++++++++++++++++
  Add2 : Sum  Inputs=++++++++++++++++++++
  Delay{,1..39} (40 alike) : Delay  DelayLength=1
  Gain : Gain  Gain=1/40
  Vol : Outport
  wires:
  Add/1 -> Gain/1
  Gain/1 -> Vol/1
  Delay36/1 -> Delay37/1, Add2/7
  Delay37/1 -> Delay38/1, Add2/8
  Delay34/1 -> Delay35/1, Add2/5
  Delay33/1 -> Delay34/1, Add2/4
  Delay20/1 -> Delay21/1, Add2/1
  Delay32/1 -> Delay33/1, Add2/3
  Add2/1 -> Add/2
  Delay35/1 -> Delay36/1, Add2/6
  Delay21/1 -> Delay32/1, Add2/2
  Delay38/1 -> Delay39/1, Add2/9
  Delay39/1 -> Delay22/1, Add2/10
  Delay31/1 -> Add2/20
  Delay19/1 -> Add1/20, Delay20/1
  Delay30/1 -> Delay31/1, Add2/19
  Delay23/1 -> Delay24/1, Add2/12
  Delay27/1 -> Delay28/1, Add2/16
  Delay24/1 -> Delay25/1, Add2/13
  Delay22/1 -> Delay23/1, Add2/11
  Delay25/1 -> Delay26/1, Add2/14
  Delay26/1 -> Delay27/1, Add2/15
  Delay29/1 -> Delay30/1, Add2/18
  Delay28/1 -> Delay29/1, Add2/17
  Delay16/1 -> Add1/17, Delay17/1
  Delay17/1 -> Add1/18, Delay18/1
  Delay14/1 -> Add1/15, Delay15/1
  Delay13/1 -> Add1/14, Delay14/1
  Delay10/1 -> Add1/11, Delay11/1
  Delay12/1 -> Add1/13, Delay13/1
  Delay15/1 -> Add1/16, Delay16/1
  Delay11/1 -> Add1/12, Delay12/1
  Delay18/1 -> Add1/19, Delay19/1
  In1/1 -> Delay/1
  Delay9/1 -> Add1/10, Delay10/1
  Delay8/1 -> Add1/9, Delay9/1
  Delay1/1 -> Add1/2, Delay2/1
  Delay5/1 -> Add1/6, Delay6/1
  Add1/1 -> Add/1
  Delay2/1 -> Add1/3, Delay3/1
  Delay/1 -> Add1/1, Delay1/1
  Delay3/1 -> Add1/4, Delay4/1
  Delay4/1 -> Add1/5, Delay5/1
  Delay7/1 -> Add1/8, Delay8/1
  Delay6/1 -> Add1/7, Delay7/1

== system EHB_speedgoat_R2020a_V1/TIF_04/CB2020_3/mean6 ==
  In1 : Inport
  Add : Sum
  Add1 : Sum  Inputs=++++++++++++++++++++
  Add2 : Sum  Inputs=++++++++++++++++++++
  Delay{,1..39} (40 alike) : Delay  DelayLength=1
  Gain : Gain  Gain=1/40
  Vol : Outport
  wires:
  Delay6/1 -> Delay7/1, Add1/7
  Delay7/1 -> Delay8/1, Add1/8
  Delay4/1 -> Delay5/1, Add1/5
  Delay3/1 -> Delay4/1, Add1/4
  Delay/1 -> Delay1/1, Add1/1
  Delay2/1 -> Delay3/1, Add1/3
  Add1/1 -> Add/1
  Delay5/1 -> Delay6/1, Add1/6
  Delay1/1 -> Delay2/1, Add1/2
  Delay8/1 -> Delay9/1, Add1/9
  Delay9/1 -> Delay10/1, Add1/10
  In1/1 -> Delay/1
  Delay18/1 -> Delay19/1, Add1/19
  Delay11/1 -> Delay12/1, Add1/12
  Delay15/1 -> Delay16/1, Add1/16
  Delay12/1 -> Delay13/1, Add1/13
  Delay10/1 -> Delay11/1, Add1/11
  Delay13/1 -> Delay14/1, Add1/14
  Delay14/1 -> Delay15/1, Add1/15
  Delay17/1 -> Delay18/1, Add1/18
  Delay16/1 -> Delay17/1, Add1/17
  Delay28/1 -> Add2/17, Delay29/1
  Delay29/1 -> Add2/18, Delay30/1
  Delay26/1 -> Add2/15, Delay27/1
  Delay25/1 -> Add2/14, Delay26/1
  Delay22/1 -> Add2/11, Delay23/1
  Delay24/1 -> Add2/13, Delay25/1
  Delay27/1 -> Add2/16, Delay28/1
  Delay23/1 -> Add2/12, Delay24/1
  Delay30/1 -> Add2/19, Delay31/1
  Delay19/1 -> Delay20/1, Add1/20
  Delay31/1 -> Add2/20
  Delay39/1 -> Add2/10, Delay22/1
  Delay38/1 -> Add2/9, Delay39/1
  Delay21/1 -> Add2/2, Delay32/1
  Delay35/1 -> Add2/6, Delay36/1
  Add2/1 -> Add/2
  Delay32/1 -> Add2/3, Delay33/1
  Delay20/1 -> Add2/1, Delay21/1
  Delay33/1 -> Add2/4, Delay34/1
  Delay34/1 -> Add2/5, Delay35/1
  Delay37/1 -> Add2/8, Delay38/1
  Delay36/1 -> Add2/7, Delay37/1
  Gain/1 -> Vol/1
  Add/1 -> Gain/1

== system EHB_speedgoat_R2020a_V1/TIF_04/CB2020_3/mean7 ==
  In1 : Inport
  Add : Sum
  Add1 : Sum  Inputs=++++++++++++++++++++
  Add2 : Sum  Inputs=++++++++++++++++++++
  Delay{,1..39} (40 alike) : Delay  DelayLength=1
  Gain : Gain  Gain=1/40
  Vol : Outport
  wires:
  Add/1 -> Gain/1
  Gain/1 -> Vol/1
  Delay36/1 -> Delay37/1, Add2/7
  Delay37/1 -> Delay38/1, Add2/8
  Delay34/1 -> Delay35/1, Add2/5
  Delay33/1 -> Delay34/1, Add2/4
  Delay20/1 -> Delay21/1, Add2/1
  Delay32/1 -> Delay33/1, Add2/3
  Add2/1 -> Add/2
  Delay35/1 -> Delay36/1, Add2/6
  Delay21/1 -> Delay32/1, Add2/2
  Delay38/1 -> Delay39/1, Add2/9
  Delay39/1 -> Delay22/1, Add2/10
  Delay31/1 -> Add2/20
  Delay19/1 -> Add1/20, Delay20/1
  Delay30/1 -> Delay31/1, Add2/19
  Delay23/1 -> Delay24/1, Add2/12
  Delay27/1 -> Delay28/1, Add2/16
  Delay24/1 -> Delay25/1, Add2/13
  Delay22/1 -> Delay23/1, Add2/11
  Delay25/1 -> Delay26/1, Add2/14
  Delay26/1 -> Delay27/1, Add2/15
  Delay29/1 -> Delay30/1, Add2/18
  Delay28/1 -> Delay29/1, Add2/17
  Delay16/1 -> Add1/17, Delay17/1
  Delay17/1 -> Add1/18, Delay18/1
  Delay14/1 -> Add1/15, Delay15/1
  Delay13/1 -> Add1/14, Delay14/1
  Delay10/1 -> Add1/11, Delay11/1
  Delay12/1 -> Add1/13, Delay13/1
  Delay15/1 -> Add1/16, Delay16/1
  Delay11/1 -> Add1/12, Delay12/1
  Delay18/1 -> Add1/19, Delay19/1
  In1/1 -> Delay/1
  Delay9/1 -> Add1/10, Delay10/1
  Delay8/1 -> Add1/9, Delay9/1
  Delay1/1 -> Add1/2, Delay2/1
  Delay5/1 -> Add1/6, Delay6/1
  Add1/1 -> Add/1
  Delay2/1 -> Add1/3, Delay3/1
  Delay/1 -> Add1/1, Delay1/1
  Delay3/1 -> Add1/4, Delay4/1
  Delay4/1 -> Add1/5, Delay5/1
  Delay7/1 -> Add1/8, Delay8/1
  Delay6/1 -> Add1/7, Delay7/1

== system EHB_speedgoat_R2020a_V1/TIF_04/CB2020_3/mean8 ==
  In1 : Inport
  Add : Sum
  Add1 : Sum  Inputs=++++++++++++++++++++
  Add2 : Sum  Inputs=++++++++++++++++++++
  Delay{,1..39} (40 alike) : Delay  DelayLength=1
  Gain : Gain  Gain=1/40
  Vol : Outport
  wires:
  Delay6/1 -> Delay7/1, Add1/7
  Delay7/1 -> Delay8/1, Add1/8
  Delay4/1 -> Delay5/1, Add1/5
  Delay3/1 -> Delay4/1, Add1/4
  Delay/1 -> Delay1/1, Add1/1
  Delay2/1 -> Delay3/1, Add1/3
  Add1/1 -> Add/1
  Delay5/1 -> Delay6/1, Add1/6
  Delay1/1 -> Delay2/1, Add1/2
  Delay8/1 -> Delay9/1, Add1/9
  Delay9/1 -> Delay10/1, Add1/10
  In1/1 -> Delay/1
  Delay18/1 -> Delay19/1, Add1/19
  Delay11/1 -> Delay12/1, Add1/12
  Delay15/1 -> Delay16/1, Add1/16
  Delay12/1 -> Delay13/1, Add1/13
  Delay10/1 -> Delay11/1, Add1/11
  Delay13/1 -> Delay14/1, Add1/14
  Delay14/1 -> Delay15/1, Add1/15
  Delay17/1 -> Delay18/1, Add1/18
  Delay16/1 -> Delay17/1, Add1/17
  Delay28/1 -> Add2/17, Delay29/1
  Delay29/1 -> Add2/18, Delay30/1
  Delay26/1 -> Add2/15, Delay27/1
  Delay25/1 -> Add2/14, Delay26/1
  Delay22/1 -> Add2/11, Delay23/1
  Delay24/1 -> Add2/13, Delay25/1
  Delay27/1 -> Add2/16, Delay28/1
  Delay23/1 -> Add2/12, Delay24/1
  Delay30/1 -> Add2/19, Delay31/1
  Delay19/1 -> Delay20/1, Add1/20
  Delay31/1 -> Add2/20
  Delay39/1 -> Add2/10, Delay22/1
  Delay38/1 -> Add2/9, Delay39/1
  Delay21/1 -> Add2/2, Delay32/1
  Delay35/1 -> Add2/6, Delay36/1
  Add2/1 -> Add/2
  Delay32/1 -> Add2/3, Delay33/1
  Delay20/1 -> Add2/1, Delay21/1
  Delay33/1 -> Add2/4, Delay34/1
  Delay34/1 -> Add2/5, Delay35/1
  Delay37/1 -> Add2/8, Delay38/1
  Delay36/1 -> Add2/7, Delay37/1
  Gain/1 -> Vol/1
  Add/1 -> Gain/1

== system EHB_speedgoat_R2020a_V1/TIF_04/CB2020_3/mean9 ==
  In1 : Inport
  Add : Sum
  Add1 : Sum  Inputs=++++++++++++++++++++
  Add2 : Sum  Inputs=++++++++++++++++++++
  Delay{,1..39} (40 alike) : Delay  DelayLength=1
  Gain : Gain  Gain=1/40
  Vol : Outport
  wires:
  Add/1 -> Gain/1
  Gain/1 -> Vol/1
  Delay36/1 -> Delay37/1, Add2/7
  Delay37/1 -> Delay38/1, Add2/8
  Delay34/1 -> Delay35/1, Add2/5
  Delay33/1 -> Delay34/1, Add2/4
  Delay20/1 -> Delay21/1, Add2/1
  Delay32/1 -> Delay33/1, Add2/3
  Add2/1 -> Add/2
  Delay35/1 -> Delay36/1, Add2/6
  Delay21/1 -> Delay32/1, Add2/2
  Delay38/1 -> Delay39/1, Add2/9
  Delay39/1 -> Delay22/1, Add2/10
  Delay31/1 -> Add2/20
  Delay19/1 -> Add1/20, Delay20/1
  Delay30/1 -> Delay31/1, Add2/19
  Delay23/1 -> Delay24/1, Add2/12
  Delay27/1 -> Delay28/1, Add2/16
  Delay24/1 -> Delay25/1, Add2/13
  Delay22/1 -> Delay23/1, Add2/11
  Delay25/1 -> Delay26/1, Add2/14
  Delay26/1 -> Delay27/1, Add2/15
  Delay29/1 -> Delay30/1, Add2/18
  Delay28/1 -> Delay29/1, Add2/17
  Delay16/1 -> Add1/17, Delay17/1
  Delay17/1 -> Add1/18, Delay18/1
  Delay14/1 -> Add1/15, Delay15/1
  Delay13/1 -> Add1/14, Delay14/1
  Delay10/1 -> Add1/11, Delay11/1
  Delay12/1 -> Add1/13, Delay13/1
  Delay15/1 -> Add1/16, Delay16/1
  Delay11/1 -> Add1/12, Delay12/1
  Delay18/1 -> Add1/19, Delay19/1
  In1/1 -> Delay/1
  Delay9/1 -> Add1/10, Delay10/1
  Delay8/1 -> Add1/9, Delay9/1
  Delay1/1 -> Add1/2, Delay2/1
  Delay5/1 -> Add1/6, Delay6/1
  Add1/1 -> Add/1
  Delay2/1 -> Add1/3, Delay3/1
  Delay/1 -> Add1/1, Delay1/1
  Delay3/1 -> Add1/4, Delay4/1
  Delay4/1 -> Add1/5, Delay5/1
  Delay7/1 -> Add1/8, Delay8/1
  Delay6/1 -> Add1/7, Delay7/1

== system EHB_speedgoat_R2020a_V1/YS5002/YS5002_M_PowerCtrl/CANDataPack_ToUDP ==
  In1 : Inport
  "Bit Packing " : xpcutilitieslib/Bit Packing   MaskBitPatterns={[7],[6],[4 5],[0:3]}  MaskPackDataType=uint8  MaskPackDataSize=[1]
      settings: SourceProductBaseCode=XP
  Bit Slice : hdlsllib/Logic and Bit Operations/Bit Slice  lidx=3  ridx=0
      settings: SourceProductBaseCode=SL
  Bus Selector : BusSelector  OutputSignals=Extended,Length,Remote,ID,Data
  "Byte Packing " : xpcutilitieslib/Byte Packing   MaskPackedDataType=uint8  MaskUnpackedDataTypes={'uint32'}  MaskAlignment=1
  "Byte Reversal " : xpcutilitieslib/Byte Reversal   numInp=1
      settings: SourceProductBaseCode=XP
  Constant1 : Constant  Value=[0 0]
  Data Type Conversion1 : DataTypeConversion  OutDataTypeStr=boolean
  Data Type Conversion2 : DataTypeConversion  OutDataTypeStr=uint8
  Data Type Conversion9 : DataTypeConversion  OutDataTypeStr=boolean
  Mux : Mux  Inputs=3
  Out1 : Outport
  wires:
  Bus Selector/5 -> Mux/3  "<Data>"
  "Bit Packing "/1 -> Mux/1  "YS5002_PowerSet"
  Bus Selector/2 -> Data Type Conversion2/1  "<Length>"
  Bus Selector/4 -> "Byte Reversal "/1  "<ID>"
  In1/1 -> Bus Selector/1
  Bus Selector/1 -> Data Type Conversion9/1  "<Extended>"
  Bus Selector/3 -> Data Type Conversion1/1  "<Remote>"
  Data Type Conversion9/1 -> "Bit Packing "/1
  "Byte Reversal "/1 -> "Byte Packing "/1
  Bit Slice/1 -> "Bit Packing "/4
  "Byte Packing "/1 -> Mux/2
  Constant1/1 -> "Bit Packing "/3
  Mux/1 -> Out1/1
  Data Type Conversion2/1 -> Bit Slice/1
  Data Type Conversion1/1 -> "Bit Packing "/2

== system EHB_speedgoat_R2020a_V1/保留/IO602/CAN Read Loop - Port 1 ==
  SampleTime : Inport
  CAN Read : speedgoatlib_IO602_4/Legacy/CAN Read  id=1  ts=-1  channel=4  messageType=CAN  canType=CAN (HS)  BusOutput=off  initValues=[602 1 -1 3 1 1 0]
      settings: SourceProductName=Simulink Real-Time: Speedgoat I/O Blockset
  CAN Unpack : canmsglib/CAN Unpack  MsgList=(none)  MsgName=CAN Msg  MsgIDType=Standard (11-bit identifier)  MsgIdentifier=100  MsgLength=8  SignalInfo={'Signal1','0','64','LE','double','Standard','0','1','0','-Inf','Inf'}  IDPort=off  TimestampPort=off  ErrorPort=off  RemotePort=off  LengthPort=off  StatusPort=off  ApplyMinMax=off
      settings: SourceProductBaseCode=ME,VN
  CAN Unpack1 : canmsglib/CAN Unpack  MsgList=(none)  MsgName=CAN Msg  MsgIDType=Standard (11-bit identifier)  MsgIdentifier=101  MsgLength=8  SignalInfo={'Signal1','0','64','LE','double','Standard','0','1','0','-Inf','Inf'}  IDPort=off  TimestampPort=off  ErrorPort=off  RemotePort=off  LengthPort=off  StatusPort=off  ApplyMinMax=off
      settings: SourceProductBaseCode=ME,VN
  CAN Unpack2 : canmsglib/CAN Unpack  MsgList=(none)  MsgName=CAN Msg  MsgIDType=Standard (11-bit identifier)  MsgIdentifier=102  MsgLength=8  SignalInfo={'Signal1','0','64','LE','double','Standard','0','1','0','-Inf','Inf'}  IDPort=off  TimestampPort=off  ErrorPort=off  RemotePort=off  LengthPort=off  StatusPort=off  ApplyMinMax=off
      settings: SourceProductBaseCode=ME,VN
  Terminator : Terminator
  While Iterator : WhileIterator  MaxIters=501  WhileBlockType=do-while
  ID100_Signal1 : Outport
  ID101_Signal1 : Outport  Port=2
  ID102_Signal1 : Outport  Port=3
  wires:
  CAN Read/2 -> CAN Unpack2/1, CAN Unpack1/1, CAN Unpack/1
  CAN Read/1 -> While Iterator/1
  CAN Unpack/1 -> ID100_Signal1/1
  CAN Unpack1/1 -> ID101_Signal1/1
  CAN Unpack2/1 -> ID102_Signal1/1
  SampleTime/1 -> Terminator/1

== system EHB_speedgoat_R2020a_V1/保留/IO602/CAN Read Loop - Port 3 ==
  SampleTime : Inport
  CAN Read : speedgoatlib_IO602_4/Legacy/CAN Read  id=1  ts=-1  channel=2  messageType=CAN  canType=CAN (HS)  BusOutput=off  initValues=[602 1 -1 1 1 1 0]
      settings: SourceProductName=Simulink Real-Time: Speedgoat I/O Blockset
  CAN Unpack : canmsglib/CAN Unpack  MsgList=(none)  MsgName=CAN Msg  MsgIDType=Standard (11-bit identifier)  MsgIdentifier=100  MsgLength=8  SignalInfo={'Signal1','0','64','LE','double','Standard','0','1','0','-Inf','Inf'}  IDPort=off  TimestampPort=off  ErrorPort=off  RemotePort=off  LengthPort=off  StatusPort=off  ApplyMinMax=off
      settings: SourceProductBaseCode=ME,VN
  CAN Unpack1 : canmsglib/CAN Unpack  MsgList=(none)  MsgName=CAN Msg  MsgIDType=Standard (11-bit identifier)  MsgIdentifier=101  MsgLength=8  SignalInfo={'Signal1','0','64','LE','double','Standard','0','1','0','-Inf','Inf'}  IDPort=off  TimestampPort=off  ErrorPort=off  RemotePort=off  LengthPort=off  StatusPort=off  ApplyMinMax=off
      settings: SourceProductBaseCode=ME,VN
  CAN Unpack2 : canmsglib/CAN Unpack  MsgList=(none)  MsgName=CAN Msg  MsgIDType=Standard (11-bit identifier)  MsgIdentifier=102  MsgLength=8  SignalInfo={'Signal1','0','64','LE','double','Standard','0','1','0','-Inf','Inf'}  IDPort=off  TimestampPort=off  ErrorPort=off  RemotePort=off  LengthPort=off  StatusPort=off  ApplyMinMax=off
      settings: SourceProductBaseCode=ME,VN
  Terminator : Terminator
  While Iterator : WhileIterator  MaxIters=501  WhileBlockType=do-while
  ID100_Signal1 : Outport
  ID101_Signal1 : Outport  Port=2
  ID102_Signal1 : Outport  Port=3
  wires:
  SampleTime/1 -> Terminator/1
  CAN Unpack2/1 -> ID102_Signal1/1
  CAN Unpack1/1 -> ID101_Signal1/1
  CAN Unpack/1 -> ID100_Signal1/1
  CAN Read/1 -> While Iterator/1
  CAN Read/2 -> CAN Unpack/1, CAN Unpack1/1, CAN Unpack2/1

== system EHB_speedgoat_R2020a_V1/保留/IO611/CAN Read Loop - Port 3 ==
  SampleTime : Inport
  CAN Read1 : speedgoatlib_IO611/Legacy/CAN/CAN Read  id=1  sampleTime=-1  portSelection=2  messageType=CAN  BusOutput=off  protl=IO611  ptIdx=1  isFDMod=1
      settings: SourceProductName=Simulink Real-Time: Speedgoat I/O Blockset
  CAN Unpack : canmsglib/CAN Unpack  MsgList=(none)  MsgName=CAN Msg  MsgIDType=Standard (11-bit identifier)  MsgIdentifier=100  MsgLength=8  SignalInfo={'Signal1','0','64','LE','double','Standard','0','1','0','-Inf','Inf'}  IDPort=off  TimestampPort=off  ErrorPort=off  RemotePort=off  LengthPort=off  StatusPort=off  ApplyMinMax=off
      settings: SourceProductBaseCode=ME,VN
  CAN Unpack1 : canmsglib/CAN Unpack  MsgList=(none)  MsgName=CAN Msg  MsgIDType=Standard (11-bit identifier)  MsgIdentifier=101  MsgLength=8  SignalInfo={'Signal1','0','64','LE','double','Standard','0','1','0','-Inf','Inf'}  IDPort=off  TimestampPort=off  ErrorPort=off  RemotePort=off  LengthPort=off  StatusPort=off  ApplyMinMax=off
      settings: SourceProductBaseCode=ME,VN
  CAN Unpack2 : canmsglib/CAN Unpack  MsgList=(none)  MsgName=CAN Msg  MsgIDType=Standard (11-bit identifier)  MsgIdentifier=102  MsgLength=8  SignalInfo={'Signal1','0','64','LE','double','Standard','0','1','0','-Inf','Inf'}  IDPort=off  TimestampPort=off  ErrorPort=off  RemotePort=off  LengthPort=off  StatusPort=off  ApplyMinMax=off
      settings: SourceProductBaseCode=ME,VN
  Terminator : Terminator
  While Iterator : WhileIterator  MaxIters=501  WhileBlockType=do-while
  ID100_Signal1 : Outport
  ID101_Signal1 : Outport  Port=2
  ID102_Signal1 : Outport  Port=3
  wires:
  SampleTime/1 -> Terminator/1
  CAN Unpack2/1 -> ID102_Signal1/1
  CAN Unpack1/1 -> ID101_Signal1/1
  CAN Unpack/1 -> ID100_Signal1/1
  CAN Read1/1 -> While Iterator/1
  CAN Read1/2 -> CAN Unpack/1, CAN Unpack1/1, CAN Unpack2/1

== system EHB_speedgoat_R2020a_V1/保留/TIF_01/YS4020_M_2 ==
  note: 每路通道4种故障类型，同时最多只能有1个为1（软件保护），当一个通道同时注入超过一种故障时，会自动清除当前通道的所有故障，恢复默认模式。
  note: Password = 0xAA
      |
      | Slot表示板卡的编号，由板卡上的拨码开关决定；
  note: FIU_SetCH: 0 无故障
      | 1 短路到KL30
      | 2 短路到KL31
      | 4 共轨
      | 8 开路
  FIU_SetCH{1..20} (20 alike) : Constant  Value=0  OutDataTypeStr=Inherit: Inherit via back propagation
  PassWord : Constant  Value=0xAA  OutDataTypeStr=uint8
  YS4020_M : Subsystem
  YS4020_M_Slot : Constant  Value=2  OutDataTypeStr=uint8
  wires:
  FIU_SetCH9/1 -> YS4020_M/9(FIU_SetCH9)  "FIU_SetCH9"
  FIU_SetCH5/1 -> YS4020_M/5(FIU_SetCH5)  "FIU_SetCH5"
  FIU_SetCH7/1 -> YS4020_M/7(FIU_SetCH7)  "FIU_SetCH7"
  FIU_SetCH4/1 -> YS4020_M/4(FIU_SetCH4)  "FIU_SetCH4"
  FIU_SetCH14/1 -> YS4020_M/14(FIU_SetCH14)  "FIU_SetCH14"
  FIU_SetCH2/1 -> YS4020_M/2(FIU_SetCH2)  "FIU_SetCH2"
  FIU_SetCH3/1 -> YS4020_M/3(FIU_SetCH3)  "FIU_SetCH3"
  FIU_SetCH13/1 -> YS4020_M/13(FIU_SetCH13)  "FIU_SetCH13"
  FIU_SetCH6/1 -> YS4020_M/6(FIU_SetCH6)  "FIU_SetCH6"
  FIU_SetCH8/1 -> YS4020_M/8(FIU_SetCH8)  "FIU_SetCH8"
  FIU_SetCH20/1 -> YS4020_M/20(FIU_SetCH20)  "FIU_SetCH20"
  FIU_SetCH12/1 -> YS4020_M/12(FIU_SetCH12)  "FIU_SetCH12"
  FIU_SetCH11/1 -> YS4020_M/11(FIU_SetCH11)  "FIU_SetCH11"
  FIU_SetCH1/1 -> YS4020_M/1(FIU_SetCH1)  "FIU_SetCH1"
  FIU_SetCH10/1 -> YS4020_M/10(FIU_SetCH10)  "FIU_SetCH10"
  FIU_SetCH17/1 -> YS4020_M/17(FIU_SetCH17)  "FIU_SetCH17"
  FIU_SetCH15/1 -> YS4020_M/15(FIU_SetCH15)  "FIU_SetCH15"
  FIU_SetCH18/1 -> YS4020_M/18(FIU_SetCH18)  "FIU_SetCH18"
  PassWord/1 -> YS4020_M/21(PassWord)  "PassWord"
  FIU_SetCH19/1 -> YS4020_M/19(FIU_SetCH19)  "FIU_SetCH19"
  FIU_SetCH16/1 -> YS4020_M/16(FIU_SetCH16)  "FIU_SetCH16"
  YS4020_M_Slot/1 -> YS4020_M/22(YS4020_M_Slot)  "YS4020_M_Slot"

== system EHB_speedgoat_R2020a_V1/保留/TIF_02/CB3012_01 ==
  G2 RES : Subsystem  mask(simucat_resistancesgenerator_g2){deviceID=0, boxNum=Box 8 (G2 Resistance Board), channel1=on, channel2=on, channel3=on, channel4=on, channel5=on, channel6=on, channel7=on, channel8=on, channel9=on, channel10=on, channel11=on, channel12=on, enableFIU=off}
      mask prompts: deviceID "Device Index:"; boxNum "Select a box:"; channel1 "1"; channel2 "2"; channel3 "3"; channel4 "4"; channel5 "5"; channel6 "6"; channel7 "7"; channel8 "8"; channel9 "9"; channel10 "10"; channel11 "11"; channel12 "12"; enableFIU "Enable FIU"
      mask help:
      | SimuCat系列电阻板卡驱动模块。
      | 功能：电阻模拟（第二代）。通道数：12
      mask TypeOptions deviceID: 0 | 1 | 2 | 3 | 4 | 5 | 6 | 7 | 8 | 9 | 10 | 11 | 12 | 13 | 14 | 15
      mask TypeOptions boxNum: Box 8 (G2 Resistance Board)
      mask DialogControl refreshButton Prompt: Refresh
      mask DialogControl refreshButton Callback: ystbx.mask.callbacks.refreshBoxList
      mask DialogControl selectChannel Prompt: Select channels:
      mask DialogControl Dummy Prompt: (Add text here)
      mask DialogControl channelSelectAll Prompt: Select All
      mask DialogControl channelSelectAll Callback: ystbx.mask.callbacks.selectAllChannels();
      mask DialogControl channelClearAll Prompt: Clear All
      mask DialogControl channelClearAll Callback: ystbx.mask.callbacks.clearAllChannels();
      mask DialogControl applyButton Prompt: Apply Modification
      mask DialogControl applyButton Callback: ystbx.mask.callbacks.maskApply();
      mask Display: disp('CB3012(G2 Resistance Board)\nresistance generator\nNetwork Device 0\nBox 8 (G2 Resistance Board)');port_label('input',1,'Res_CH1');port_label('input',2,'Res_CH2');port_label('input',3,'Res_CH3');port_label('input',4,'Res_CH4');port_label('input',5,'Res_CH5');port_label('input',6,'Res_CH6');port_label('input',7,'Res_CH7');port_label('input',8,'Res_CH8');port_label('input',9,'Res_CH9');port_label('input',10,'Res_CH10');port_label('input',11,'Res_CH11');port_label('input',12,'Res_CH12');
  Res2Cmd : Subsystem
  Res2Cmd1 : Subsystem
  Res2Cmd10 : Subsystem
  Res2Cmd11 : Subsystem
  Res2Cmd2 : Subsystem
  Res2Cmd3 : Subsystem
  Res2Cmd4 : Subsystem
  Res2Cmd5 : Subsystem
  Res2Cmd6 : Subsystem
  Res2Cmd7 : Subsystem
  Res2Cmd8 : Subsystem
  Res2Cmd9 : Subsystem
  Res_CH1 : Constant  Value=1000000  OutDataTypeStr=Inherit: Inherit via back propagation
  Res_CH{2..6,8..12} (10 alike) : Constant  Value=100000  OutDataTypeStr=Inherit: Inherit via back propagation
  Res_CH7 : Constant  Value=1000000  OutDataTypeStr=Inherit: Inherit via back propagation
  wires:
  Res_CH8/1 -> Res2Cmd7/1(ResVal)
  Res_CH9/1 -> Res2Cmd8/1(ResVal)
  Res_CH7/1 -> Res2Cmd6/1(ResVal)
  Res_CH12/1 -> Res2Cmd11/1(ResVal)
  Res_CH10/1 -> Res2Cmd9/1(ResVal)
  Res_CH4/1 -> Res2Cmd3/1(ResVal)
  Res_CH3/1 -> Res2Cmd2/1(ResVal)
  Res_CH11/1 -> Res2Cmd10/1(ResVal)
  Res_CH5/1 -> Res2Cmd4/1(ResVal)
  Res_CH2/1 -> Res2Cmd1/1(ResVal)
  Res_CH1/1 -> Res2Cmd/1(ResVal)
  Res_CH6/1 -> Res2Cmd5/1(ResVal)
  Res2Cmd/1(CmdVal) -> G2 RES/1(Res_CH1)
  Res2Cmd1/1(CmdVal) -> G2 RES/2(Res_CH2)
  Res2Cmd2/1(CmdVal) -> G2 RES/3(Res_CH3)
  Res2Cmd3/1(CmdVal) -> G2 RES/4(Res_CH4)
  Res2Cmd4/1(CmdVal) -> G2 RES/5(Res_CH5)
  Res2Cmd5/1(CmdVal) -> G2 RES/6(Res_CH6)
  Res2Cmd6/1(CmdVal) -> G2 RES/7(Res_CH7)
  Res2Cmd7/1(CmdVal) -> G2 RES/8(Res_CH8)
  Res2Cmd8/1(CmdVal) -> G2 RES/9(Res_CH9)
  Res2Cmd9/1(CmdVal) -> G2 RES/10(Res_CH10)
  Res2Cmd10/1(CmdVal) -> G2 RES/11(Res_CH11)
  Res2Cmd11/1(CmdVal) -> G2 RES/12(Res_CH12)

== system EHB_speedgoat_R2020a_V1/保留/TIF_03/CB1032_3 ==
  note: CB1032_03配置为PWM OUT
  DIO : Subsystem
  PWM : Subsystem

== system EHB_speedgoat_R2020a_V1/保留/TIF_03/CB1032_4 ==
  note: CB1032_04配置为PWM IN
  DIO : Subsystem
  PWM : Subsystem

== system EHB_speedgoat_R2020a_V1/保留/TIF_06/CB1032_1 ==
  note: CB1032_01配置为DO
  DIO : Subsystem
  PWM : Subsystem

== system EHB_speedgoat_R2020a_V1/保留/TIF_06/CB1032_2 ==
  note: CB1032_02配置为DI
  DIO : Subsystem
  PWM : Subsystem

== system EHB_speedgoat_R2020a_V1/保留/TIF_06/YS4020_M_1 ==
  note: 每路通道4种故障类型，同时最多只能有1个为1（软件保护），当一个通道同时注入超过一种故障时，会自动清除当前通道的所有故障，恢复默认模式。
  note: Password = 0xAA
      |
      | Slot表示板卡的编号，由板卡上的拨码开关决定；
  note: FIU_SetCH: 0 无故障
      | 1 短路到KL30
      | 2 短路到KL31
      | 4 共轨
      | 8 开路
  FIU_SetCH{1..20} (20 alike) : Constant  Value=0  OutDataTypeStr=Inherit: Inherit via back propagation
  PassWord : Constant  Value=0xAA  OutDataTypeStr=uint8
  YS4020_M : Subsystem
  YS4020_M_Slot : Constant  OutDataTypeStr=uint8
  wires:
  FIU_SetCH2/1 -> YS4020_M/2(FIU_SetCH2)  "FIU_SetCH2"
  FIU_SetCH15/1 -> YS4020_M/15(FIU_SetCH15)  "FIU_SetCH15"
  FIU_SetCH7/1 -> YS4020_M/7(FIU_SetCH7)  "FIU_SetCH7"
  FIU_SetCH14/1 -> YS4020_M/14(FIU_SetCH14)  "FIU_SetCH14"
  FIU_SetCH5/1 -> YS4020_M/5(FIU_SetCH5)  "FIU_SetCH5"
  FIU_SetCH9/1 -> YS4020_M/9(FIU_SetCH9)  "FIU_SetCH9"
  FIU_SetCH10/1 -> YS4020_M/10(FIU_SetCH10)  "FIU_SetCH10"
  FIU_SetCH16/1 -> YS4020_M/16(FIU_SetCH16)  "FIU_SetCH16"
  YS4020_M_Slot/1 -> YS4020_M/22(YS4020_M_Slot)  "YS4020_M_Slot"
  FIU_SetCH6/1 -> YS4020_M/6(FIU_SetCH6)  "FIU_SetCH6"
  FIU_SetCH1/1 -> YS4020_M/1(FIU_SetCH1)  "FIU_SetCH1"
  FIU_SetCH12/1 -> YS4020_M/12(FIU_SetCH12)  "FIU_SetCH12"
  FIU_SetCH17/1 -> YS4020_M/17(FIU_SetCH17)  "FIU_SetCH17"
  FIU_SetCH18/1 -> YS4020_M/18(FIU_SetCH18)  "FIU_SetCH18"
  FIU_SetCH8/1 -> YS4020_M/8(FIU_SetCH8)  "FIU_SetCH8"
  FIU_SetCH13/1 -> YS4020_M/13(FIU_SetCH13)  "FIU_SetCH13"
  FIU_SetCH3/1 -> YS4020_M/3(FIU_SetCH3)  "FIU_SetCH3"
  PassWord/1 -> YS4020_M/21(PassWord)  "PassWord"
  FIU_SetCH19/1 -> YS4020_M/19(FIU_SetCH19)  "FIU_SetCH19"
  FIU_SetCH11/1 -> YS4020_M/11(FIU_SetCH11)  "FIU_SetCH11"
  FIU_SetCH20/1 -> YS4020_M/20(FIU_SetCH20)  "FIU_SetCH20"
  FIU_SetCH4/1 -> YS4020_M/4(FIU_SetCH4)  "FIU_SetCH4"
